simulink library "HDL_ieee_8021513"  (R2024a)
settings: Solver=FixedStepDiscrete  StartTime=0.0  StopTime=10.0  RelTol=1e-3
undefined symbols (not defined in the file): Add, axiWidth, CONST, fs, peakDetectorThreshold, peakDetectorWindow, QAM, Shift
libraries: hdlsllib x199, $bdroot x91, whdlutilities x34, whdledac x9, simulink x8, whdlmod x6, dspsigops x5, dsphdlfiltering2 x4, embreciprocals x3, dsphdlsigops2 x2, commhdlcrc x2, dspstat3 x2
(part 5 of 6)

== system HDL_ieee_8021513/full_tx/new_frame_rate_conversion ==
  note: Description:
      | This block "extends" the "end" signal 4 clock cycles, to ensure that the "end" signal can be sampled by the rate transition block.
      | (Otherwise, the "end" signal would be "on" only 1/4th of a cycle, and it can't be ensured that it will be read).
  ctrl_in : Inport
  Delay2 : Delay  DelayLength=1  InitialCondition=0  UseCircularBuffer=on
  Delay3 : Delay  DelayLength=1  InitialCondition=0  UseCircularBuffer=on
  Delay4 : Delay  DelayLength=1  InitialCondition=0  UseCircularBuffer=on
  Logical Operator : Logic  Operator=OR  Inputs=4  IconShape=distinctive  AllPortsSameDT=off  OutDataTypeStr=boolean
  Rate Transition2 : RateTransition  OutPortSampleTime=4/CONST.fPHY
  Sample Control Bus Selector1 : whdlutilities/Sample Control Bus Selector  OutputSignals=start,end,valid
  State Control : StateControl  StateControl=Synchronous
  Terminator2 : Terminator
  Terminator3 : Terminator
  new_frame : Outport  VectorParamsAs1DForOutWhenUnconnected=off
  wires:
  Logical Operator/1 -> Rate Transition2/1
  Sample Control Bus Selector1/3 -> Terminator2/1  "<valid>"
  Delay2/1 -> Logical Operator/2, Delay3/1
  Delay3/1 -> Logical Operator/3, Delay4/1
  Sample Control Bus Selector1/2 -> Logical Operator/1, Delay2/1  "<end>"
  Delay4/1 -> Logical Operator/4
  Sample Control Bus Selector1/1 -> Terminator3/1  "<start>"
  ctrl_in/1 -> Sample Control Bus Selector1/1
  Rate Transition2/1 -> new_frame/1

== system HDL_ieee_8021513/full_tx/new_frame_rate_conversion1 ==
  note: Description:
      | This block "extends" the "end" signal 8 clock cycles, to ensure that the "end" signal can be sampled by the rate transition block.
      | (Otherwise, the "end" signal would be "on" only 1/4th of a cycle, and it can't be ensured that it will be read).
  ctrl_in : Inport
  Delay{1..7} (7 alike) : Delay  DelayLength=1  InitialCondition=0  UseCircularBuffer=on
  Logical Operator : Logic  Operator=OR  Inputs=8  IconShape=distinctive  AllPortsSameDT=off  OutDataTypeStr=boolean
  Rate Transition2 : RateTransition  OutPortSampleTime=4/CONST.fPHY
  Sample Control Bus Selector1 : whdlutilities/Sample Control Bus Selector  OutputSignals=start,end,valid
  State Control : StateControl  StateControl=Synchronous
  Terminator2 : Terminator
  Terminator3 : Terminator
  new_frame : Outport  VectorParamsAs1DForOutWhenUnconnected=off
  wires:
  Logical Operator/1 -> Rate Transition2/1
  Sample Control Bus Selector1/3 -> Terminator2/1  "<valid>"
  Delay2/1 -> Logical Operator/2, Delay3/1
  Delay3/1 -> Logical Operator/3, Delay4/1
  Sample Control Bus Selector1/2 -> Logical Operator/1, Delay2/1  "<end>"
  Delay4/1 -> Logical Operator/8, Delay1/1
  Sample Control Bus Selector1/1 -> Terminator3/1  "<start>"
  ctrl_in/1 -> Sample Control Bus Selector1/1
  Rate Transition2/1 -> new_frame/1
  Delay1/1 -> Logical Operator/7, Delay5/1
  Delay5/1 -> Logical Operator/6, Delay6/1
  Delay6/1 -> Logical Operator/5, Delay7/1
  Delay7/1 -> Logical Operator/4

== system HDL_ieee_8021513/full_tx/store_frame_in_ram ==
  preamble : Inport
  preamble_valid : Inport  Port=2
  channel : Inport  Port=3
  channel_valid : Inport  Port=4
  header : Inport  Port=5
  header_valid : Inport  Port=6
  payload : Inport  Port=7
  payload_valid : Inport  Port=8
  payload_len : Inport  Port=9
  bits_per_subcarrier : Inport  Port=10
  cp_len_in : Inport  Port=11
  ready : Inport  Port=12
  Delay{,1..5} (6 alike) : Delay  DelayLength=1  InitialCondition=0  UseCircularBuffer=on
  Delay6 : Delay  DelayLength=4  InitialCondition=0  UseCircularBuffer=on
  Simple Dual Port RAM : hdlsllib/HDL RAMs/Simple Dual Port RAM  ram_size=CONST.txRAMAddressBitWidth
  State Control : StateControl  StateControl=Synchronous
  read_frame_from_ram : Subsystem
  write_frame_to_ram : Subsystem
  data_out : Outport
  valid_out : Outport  Port=2
  bits_per_subcarrier_out : Outport  Port=3
  init : Outport  Port=4
  new : Outport  Port=5
  cp_len : Outport  Port=6
  new_psdu : Outport  Port=7  VectorParamsAs1DForOutWhenUnconnected=off
  wires:
  Delay6/1 -> Delay5/1
  Delay5/1 -> new_psdu/1
  ready/1 -> read_frame_from_ram/5(ready)
  Delay4/1 -> cp_len/1
  Delay3/1 -> new/1
  Delay2/1 -> init/1
  Delay1/1 -> bits_per_subcarrier_out/1
  Delay/1 -> valid_out/1
  read_frame_from_ram/3(bits_per_subcarrier_out) -> Delay1/1
  read_frame_from_ram/4(init) -> Delay2/1
  read_frame_from_ram/6(cp_len) -> Delay4/1
  read_frame_from_ram/1(rd_addr) -> Simple Dual Port RAM/4  "new_rd_addr"
  bits_per_subcarrier/1 -> read_frame_from_ram/3(bits_per_subcarrier)
  header/1 -> write_frame_to_ram/5(header)
  write_frame_to_ram/1(write_data) -> Simple Dual Port RAM/1  "new_din"
  write_frame_to_ram/4(end) -> read_frame_from_ram/1(start_reading), Delay6/1
  cp_len_in/1 -> read_frame_from_ram/4(cp_len_in)
  write_frame_to_ram/3(we) -> Simple Dual Port RAM/3  "new_we"
  preamble/1 -> write_frame_to_ram/1(preamble)
  channel_valid/1 -> write_frame_to_ram/4(channel_valid)
  payload/1 -> write_frame_to_ram/7(payload)
  Simple Dual Port RAM/1 -> data_out/1
  read_frame_from_ram/5(new) -> Delay3/1  "new_new"
  write_frame_to_ram/5(ram_size) -> read_frame_from_ram/2(ram_size)
  preamble_valid/1 -> write_frame_to_ram/2(preamble_valid)
  payload_len/1 -> write_frame_to_ram/9(payload_len)
  channel/1 -> write_frame_to_ram/3(channel)
  write_frame_to_ram/2(wr_addr) -> Simple Dual Port RAM/2  "new_wr_addr"
  read_frame_from_ram/2(valid_out) -> Delay/1  "valid_new"
  payload_valid/1 -> write_frame_to_ram/8(payload_valid)
  header_valid/1 -> write_frame_to_ram/6(header_valid)

== system HDL_ieee_8021513/ldpc_encoder/output_selector ==
  codeRate : Inport
  blockSize : Inport  Port=2
  Buffer1 : $bdroot/Buffer  SystemSampleTime=-1  VariantActivationTime=update diagram  AllowFlexibleInterface=on  Latency=0  AutoFrameSizeCalculation=off
  Demux2 : Demux  Outputs=2
  Demux3 : Demux  Outputs=3
  Logical Operator3 : Logic  IconShape=distinctive  AllPortsSameDT=off  OutDataTypeStr=boolean
  Logical Operator5 : Logic  Operator=OR  IconShape=distinctive  AllPortsSameDT=off  OutDataTypeStr=boolean
  Logical Operator6 : Logic  IconShape=distinctive  AllPortsSameDT=off  OutDataTypeStr=boolean
  Logical Operator7 : Logic  Operator=NOT  IconShape=distinctive  AllPortsSameDT=off  OutDataTypeStr=boolean
  Terminator1 : Terminator
  m2 : Outport  VectorParamsAs1DForOutWhenUnconnected=off
  m1 : Outport  Port=2  VectorParamsAs1DForOutWhenUnconnected=off
  m0 : Outport  Port=3  VectorParamsAs1DForOutWhenUnconnected=off
  wires:
  Buffer1/1 -> m0/1  "Out0"
  Logical Operator6/1 -> m1/1  "Out1"
  codeRate/1 -> Demux3/1
  blockSize/1 -> Demux2/1
  Demux2/1 -> Buffer1/1  "K0"
  Demux3/1 -> Logical Operator3/2, Logical Operator7/1  "R0"
  Logical Operator5/1 -> m2/1  "Out2"
  Logical Operator7/1 -> Logical Operator6/1
  Demux3/2 -> Logical Operator6/2, Logical Operator3/1  "R1"
  Demux2/2 -> Terminator1/1  "K1"
  Logical Operator3/1 -> Logical Operator5/1
  Demux3/3 -> Logical Operator5/2  "R2"

== system HDL_ieee_8021513/ofdm_separator/wait_for_header ==
  note: Store payload OFDM symbols until header parameters are known (cyclic prefix has to be known before demodulating the OFDM symbol)
  note: The RAM value should be large enough to wait for the header to be processed.
      | Th e LDPC decoder of the header has a delay > 2500, so a value of 3000 is chosen for an extra margin.
  data_in : Inport
  header_ready : Inport  Port=2
  valid_payload : Inport  Port=3
  zero_payload : Inport  Port=4
  one_payload : Inport  Port=5
  ofdm_samples : Inport  Port=6
  AND : Logic  IconShape=distinctive  AllPortsSameDT=off  OutDataTypeStr=boolean
  Delay12 : Delay  DelayLength=1  InitialCondition=0  UseCircularBuffer=on
  Delay13 : Delay  DelayLength=1  InitialCondition=0  UseCircularBuffer=on
  Delay14 : Delay  DelayLength=1  InitialCondition=0  UseCircularBuffer=on
  HDL Counter : hdlsllib/Sources/HDL Counter  CountType=Free running  CountInit=0  CountStep=1  CountMax=25  CountFromType=Initial value  CountFrom=0  CountResetPort=on  CountLoadPort=off  CountEnbPort=on  CountDirPort=off  CountHitOutputPort=off  CountDataType=Unsigned  CountWordLen=16  CountFracLen=0  CountSampTime=1
  HDL FIFO : hdlsllib/HDL RAMs/HDL FIFO  fifo_size=CONST.FIFOOFDMSize  mode=Classic  ratio=1  push_msg=Error  pop_msg=Error  show_empty=on  show_full=off  show_num=on  LabelModeActiveChoice_Mode=Classic  rst_port=on
  Logical Operator1 : Logic  Operator=OR  Inputs=3  IconShape=distinctive  AllPortsSameDT=off  OutDataTypeStr=boolean
  NOT : Logic  Operator=NOT  IconShape=distinctive  AllPortsSameDT=off  OutDataTypeStr=boolean
  OR : Logic  Operator=OR  IconShape=distinctive  AllPortsSameDT=off  OutDataTypeStr=boolean
  OR2 : Logic  Operator=OR  IconShape=distinctive  AllPortsSameDT=off  OutDataTypeStr=boolean
  Relational Operator : RelationalOperator  Operator===  OutDataTypeStr=boolean  RndMeth=Simplest  InputSameDT=off
  Switch : Switch  Criteria=u2 ~= 0  SaturateOnIntegerOverflow=off  InputSameDT=off
  Switch3 : Switch  Criteria=u2 ~= 0  SaturateOnIntegerOverflow=off  InputSameDT=off
  Terminator : Terminator
  Unit Delay : UnitDelay  SampleTime=-1  HasFrameUpgradeWarning=on
  rising_edge_detector : $bdroot/rising_edge_detector  SystemSampleTime=-1  VariantActivationTime=update diagram  AllowFlexibleInterface=on  Latency=0  AutoFrameSizeCalculation=off
  rising_edge_detector1 : $bdroot/rising_edge_detector  SystemSampleTime=-1  VariantActivationTime=update diagram  AllowFlexibleInterface=on  Latency=0  AutoFrameSizeCalculation=off
  data_out : Outport
  valid_payload_out : Outport  Port=2
  wires:
  Delay13/1 -> HDL FIFO/2
  data_in/1 -> Switch3/3, Delay12/1
  Delay12/1 -> HDL FIFO/1
  valid_payload/1 -> Delay13/1, rising_edge_detector1/1
  Switch3/1 -> data_out/1
  HDL FIFO/2 -> [empty]
  HDL FIFO/1 -> Switch3/1
  rising_edge_detector1/1 -> OR/1
  zero_payload/1 -> OR/2
  HDL FIFO/3 -> Terminator/1  "fifo_ofdm"
  [empty] -> rising_edge_detector/1
  rising_edge_detector/1 -> Logical Operator1/1
  Unit Delay/1 -> Switch/3
  Switch/1 -> Delay14/1, HDL FIFO/3, Unit Delay/1  "pop"
  Logical Operator1/1 -> Switch/2
  header_ready/1 -> HDL Counter/1, Switch/1, Logical Operator1/2
  HDL Counter/1 -> Relational Operator/1  "count"
  ofdm_samples/1 -> Relational Operator/2
  OR/1 -> OR2/1
  Relational Operator/1 -> OR2/2, NOT/1, Logical Operator1/3  "hit_zero"
  OR2/1 -> HDL FIFO/4
  one_payload/1 -> HDL Counter/2
  AND/1 -> Switch3/2, valid_payload_out/1
  Delay14/1 -> AND/1
  NOT/1 -> AND/2

== system HDL_ieee_8021513/ofdm_symbol_sync/find_peak ==
  data_in : Inport
  M_in : Inport  Port=2
  Compare To Constant : hdlsllib/Logic and Bit Operations/Compare To Constant  relop=>  const=CONST.peakDetectorThreshold  OutDataTypeStr=boolean
  Constant : Constant  Value=0  OutDataTypeStr=Inherit: Inherit via back propagation  SampleTime=-1
  Delay{,1..4} (5 alike) : Delay  DelayLength=1  InitialCondition=0  UseCircularBuffer=on
  Delay5 : Delay  DelayLength=CONST.peakDetectorWindow-1  InitialCondition=0  UseCircularBuffer=on
  HDL Counter : hdlsllib/Sources/HDL Counter  CountType=Count limited  CountInit=0  CountStep=1  CountMax=CONST.peakDetectorWindow-1  CountFromType=Initial value  CountFrom=0  CountResetPort=on  CountLoadPort=off  CountEnbPort=on  CountDirPort=off  CountHitOutputPort=on  CountDataType=Unsigned  CountWordLen=nextpow2(CONST.peakDetectorWindow)  CountFracLen=0  CountSampTime=1
  OR : Logic  Operator=OR  IconShape=distinctive  AllPortsSameDT=off  OutDataTypeStr=boolean
  OR1 : Logic  Operator=OR  IconShape=distinctive  AllPortsSameDT=off  OutDataTypeStr=boolean
  Relational Operator : RelationalOperator  Operator=>  OutDataTypeStr=boolean  InputSameDT=off
  Switch : Switch  Criteria=u2 ~= 0  SaturateOnIntegerOverflow=off
  Switch1 : Switch  Criteria=u2 ~= 0  SaturateOnIntegerOverflow=off
  Switch2 : Switch  Criteria=u2 ~= 0  SaturateOnIntegerOverflow=off  InputSameDT=off
  Terminator : Terminator
  Unit Delay : UnitDelay  SampleTime=-1  HasFrameUpgradeWarning=on
  Unit Delay1 : UnitDelay  SampleTime=-1  HasFrameUpgradeWarning=on
  data_out : Outport  VectorParamsAs1DForOutWhenUnconnected=off
  peak_sync : Outport  Port=2  VectorParamsAs1DForOutWhenUnconnected=off
  wires:
  M_in/1 -> Switch1/1, Compare To Constant/1  "data_in"
  Unit Delay/1 -> Switch/3
  Switch/1 -> Unit Delay/1, Relational Operator/2  "peak(i)"
  Relational Operator/1 -> HDL Counter/1, Delay3/1  "new_peak"
  Switch1/1 -> Delay2/1  "peak(i+1)"
  Constant/1 -> Switch1/3
  Unit Delay1/1 -> Switch2/3
  Switch2/1 -> Unit Delay1/1, HDL Counter/2  "en"
  HDL Counter/2 -> Delay1/1, peak_sync/1
  OR/1 -> Switch2/2
  [new_peak] -> OR/2
  [peak_found] -> OR/1
  HDL Counter/1 -> Terminator/1
  Delay/1 -> Switch/1
  Delay1/1 -> [peak_found]  "peak_found"
  OR1/1 -> Switch/2
  [new_peak] -> OR1/1
  [peak_found] -> OR1/2
  Delay3/1 -> [new_peak], Switch2/1
  Compare To Constant/1 -> Switch1/2
  Delay2/1 -> Delay/1, Relational Operator/1
  data_in/1 -> Delay4/1
  Delay4/1 -> Delay5/1
  Delay5/1 -> data_out/1

== system HDL_ieee_8021513/ofdm_symbol_sync/m_cox ==
  note: Delay of m_cox = delay blocks + delay divider + delay_10_preambles_symbols
      | Delay of m_cox = 12 + 47 + 2580
  data_in : Inport
  Compare To Constant : hdlsllib/Logic and Bit Operations/Compare To Constant  relop=>=  const=1  OutDataTypeStr=boolean
  Constant : Constant  OutDataTypeStr=boolean  SampleTime=-1
  Constant1 : Constant  OutDataTypeStr=Inherit: Inherit via back propagation  SampleTime=-1
  Data Type Conversion : DataTypeConversion  OutDataTypeStr=CONST.rxPDataType  SaturateOnIntegerOverflow=off  RndMeth=Floor
  Data Type Conversion1 : DataTypeConversion  OutDataTypeStr=CONST.rxOFDMSSInputDataType  SaturateOnIntegerOverflow=off  RndMeth=Floor
  Data Type Conversion2 : DataTypeConversion  OutDataTypeStr=fixdt(0, CONST.rxRWordLength, CONST.rxRFractionLength)  SaturateOnIntegerOverflow=off  RndMeth=Floor
  Data Type Conversion3 : DataTypeConversion  OutDataTypeStr=fixdt(0, CONST.rxRWordLength, CONST.rxRFractionLength)  SaturateOnIntegerOverflow=off  RndMeth=Floor
  Delay1 : Delay  DelayLength=CONST.rxRDividerDelay  InitialCondition=0  UseCircularBuffer=on
  Delay4 : Delay  DelayLength=(CONST.N+CONST.preambleCyclicPrefixLen)*10+12+CONST.rxRDividerDelay  InitialCondition=0  UseCircularBuffer=on
  Real Divide HDL Optimized : embreciprocals/Real Divide HDL Optimized  OutputType=CONST.rxMDataType
      settings: LibrarySourceBlock=embeddedMatrixLib/Math Operations/Real Divide HDL Optimized
  Switch : Switch  Criteria=u2 ~= 0  SaturateOnIntegerOverflow=off  InputSameDT=off
  Terminator : Terminator
  calculate_P : Subsystem
  calculate_R : Subsystem
  data_out : Outport  VectorParamsAs1DForOutWhenUnconnected=off
  M(d) : Outport  Port=2  VectorParamsAs1DForOutWhenUnconnected=off
  P(d) : Outport  Port=3  VectorParamsAs1DForOutWhenUnconnected=off
  wires:
  Data Type Conversion1/1 -> calculate_P/1(r(d)), calculate_R/1(r(d))
  Data Type Conversion3/1 -> Real Divide HDL Optimized/2
  Data Type Conversion2/1 -> Real Divide HDL Optimized/1
  data_in/1 -> Delay4/1, Data Type Conversion1/1
  Data Type Conversion/1 -> Delay1/1
  Constant/1 -> Real Divide HDL Optimized/3
  calculate_P/1(|P(d)|2) -> Data Type Conversion2/1  "p_sig"
  Real Divide HDL Optimized/1 -> M(d)/1  "M"
  Delay1/1 -> P(d)/1
  Delay4/1 -> data_out/1
  calculate_P/2(P(d)) -> Data Type Conversion/1  "p_pelado"
  Real Divide HDL Optimized/2 -> Terminator/1
  Constant1/1 -> Switch/3
  Compare To Constant/1 -> Switch/2
  Switch/1 -> Data Type Conversion3/1
  calculate_R/1(Rf2) -> Switch/1, Compare To Constant/1  "r_sig"

== system HDL_ieee_8021513/ofdm_symbol_sync/phase_offset_calculator ==
  peak_sync : Inport
  P(d) : Inport  Port=2
  Complex to Magnitude-Angle : dsphdlmathfun2/Complex to Magnitude-Angle  NumIterationsSource=Auto  NumIterations=10  OutputFormat=Angle  AngleFormat=Normalized  ScaleOutput=off  ScalingMethod=Shift-Add  SimulateUsing=Code generation
  Data Type Conversion : DataTypeConversion  OutDataTypeStr=CONST.rxPhaseDataType  SaturateOnIntegerOverflow=off  RndMeth=Floor
  Delay2 : Delay  InitialCondition=0  UseCircularBuffer=on
  Delay3 : Delay  InitialCondition=0  UseCircularBuffer=on
  Switch : Switch  Criteria=u2 ~= 0  SaturateOnIntegerOverflow=off  InputSameDT=off
  Unit Delay : UnitDelay  SampleTime=-1  HasFrameUpgradeWarning=on
  frequency_offset : Outport
  wires:
  Data Type Conversion/1 -> Delay2/1
  Switch/1 -> Unit Delay/1, frequency_offset/1
  Unit Delay/1 -> Switch/3
  Delay2/1 -> Switch/1
  Delay3/1 -> Switch/2
  Complex to Magnitude-Angle/1 -> Data Type Conversion/1
  P(d)/1 -> Complex to Magnitude-Angle/1
  peak_sync/1 -> Complex to Magnitude-Angle/2
  Complex to Magnitude-Angle/2 -> Delay3/1

== system HDL_ieee_8021513/peak_detector/local_peak ==
  index : Inport
  dataIn : Inport  Port=2
  AND : Logic  IconShape=distinctive  AllPortsSameDT=off  OutDataTypeStr=boolean
  AND1 : Logic  IconShape=distinctive  AllPortsSameDT=off  OutDataTypeStr=boolean
  AND2 : Logic  IconShape=distinctive  AllPortsSameDT=off  OutDataTypeStr=boolean
  Delay{,1..5} (6 alike) : Delay  DelayLength=1  InitialCondition=0  UseCircularBuffer=on
  HDL Counter : hdlsllib/Sources/HDL Counter  CountType=Count limited  CountInit=0  CountStep=1  CountMax=peakDetectorWindow-1  CountFromType=Initial value  CountFrom=0  CountResetPort=on  CountLoadPort=off  CountEnbPort=on  CountDirPort=off  CountHitOutputPort=on  CountDataType=Unsigned  CountWordLen=nextpow2(peakDetectorWindow+1)  CountFracLen=0  CountSampTime=-1
  NOT : Logic  Operator=NOT  IconShape=distinctive  AllPortsSameDT=off  OutDataTypeStr=boolean
  OR : Logic  Operator=OR  IconShape=distinctive  AllPortsSameDT=off  OutDataTypeStr=boolean
  OR1 : Logic  Operator=OR  IconShape=distinctive  AllPortsSameDT=off  OutDataTypeStr=boolean
  OR2 : Logic  Operator=OR  IconShape=distinctive  AllPortsSameDT=off  OutDataTypeStr=boolean
  Relational Operator : RelationalOperator  OutDataTypeStr=boolean  RndMeth=Simplest  InputSameDT=off
  Switch : Switch  Criteria=u2 ~= 0  SaturateOnIntegerOverflow=off  InputSameDT=off
  Switch1 : Switch  Criteria=u2 ~= 0  SaturateOnIntegerOverflow=off  InputSameDT=off
  Terminator : Terminator
  Unit Delay : UnitDelay  SampleTime=-1  HasFrameUpgradeWarning=on
  Unit Delay1 : UnitDelay  SampleTime=-1  HasFrameUpgradeWarning=on
  peak_sync : Outport
  wires:
  HDL Counter/1 -> Terminator/1  "count"
  Unit Delay/1 -> Switch/3
  Switch/1 -> Relational Operator/2, Unit Delay/1  "dataIn(indexes(i)"
  Unit Delay1/1 -> Switch1/3
  Switch1/1 -> HDL Counter/2, Delay3/1, Unit Delay1/1  "count_enable"
  OR/1 -> Delay4/1
  dataIn/1 -> Relational Operator/1, Delay1/1
  index/1 -> AND1/1  "input"
  Delay4/1 -> Switch1/2  "open"
  Delay5/1 -> Switch1/1  "new_index"
  Delay/1 -> Switch/2
  Delay1/1 -> Switch/1
  Relational Operator/1 -> [higher]
  NOT/1 -> AND1/2
  AND1/1 -> [new_peak], OR1/1
  OR1/1 -> Delay2/1  "rst"
  AND2/1 -> OR1/2
  AND/1 -> OR2/1
  OR2/1 -> Delay/1
  [en] -> NOT/1
  [en] -> AND2/1
  [en] -> AND/1
  Delay3/1 -> [en]
  [higher] -> AND/2
  [higher] -> AND2/2
  [peak_found] -> OR/2
  HDL Counter/2 -> peak_sync/1, [peak_found]  "counter_hit"
  [new_peak] -> Delay5/1
  [new_peak] -> OR/1
  [new_peak] -> OR2/2
  Delay2/1 -> HDL Counter/1  "new_index"

== system HDL_ieee_8021513/peak_detector/s1_index ==
  dataIn : Inport
  Add : Sum
  Bit Shift : hdlsllib/Logic and Bit Operations/Bit Shift  mode=Shift Right Arithmetic  N=1
  Compare To Constant : hdlsllib/Logic and Bit Operations/Compare To Constant  relop=>  const=peakDetectorThreshold  OutDataTypeStr=boolean
  Delay : Delay  DelayLength=peakDetectorWindow  InitialCondition=0  UseCircularBuffer=on
  Delay{1..5} (5 alike) : Delay  DelayLength=1  InitialCondition=0  UseCircularBuffer=on
  Minimum : dspstat3/Minimum  operation=minimum  fcn=Value  indexBase=Zero  operateOver=Each column  Dimension=1  InputProcessing=Columns as channels (frame based)  reset=None  roiEnable=off  roiType=Rectangles  roiPortion=Entire ROI  roiOutput=Individual statistics for each ROI  roiFlag=off  roundingMode=Floor  overflowMode=off
      settings: LibrarySourceBlock=dsphdlsupportstat/Minimum
  Minimum1 : dspstat3/Minimum  operation=minimum  fcn=Value  indexBase=Zero  operateOver=Each column  Dimension=1  InputProcessing=Columns as channels (frame based)  reset=None  roiEnable=off  roiType=Rectangles  roiPortion=Entire ROI  roiOutput=Individual statistics for each ROI  roiFlag=off  roundingMode=Floor  overflowMode=off
      settings: LibrarySourceBlock=dsphdlsupportstat/Minimum
  Tapped Delay : simulink/Discrete/Tapped Delay  vinit=0.0  samptime=-1  NumDelays=peakDetectorWindow  DelayOrder=Oldest  includeCurrent=off
  Tapped Delay1 : simulink/Discrete/Tapped Delay  vinit=0.0  samptime=-1  NumDelays=peakDetectorWindow  DelayOrder=Oldest  includeCurrent=off
  indexes : Outport
  Output : Outport  Port=2
  wires:
  dataIn/1 -> Tapped Delay/1, Delay/1  "x(i+peakDetectorWindow+1)"
  Delay/1 -> Delay2/1  "x(i+1)"
  Tapped Delay/1 -> Minimum/1  "x(i+1:i+peakDetectorWindow)"
  Tapped Delay1/1 -> Minimum1/1  "x(i-peakDetectorWindow:i-1)"
  Minimum/1 -> Add/1  "xmin_new"
  Minimum1/1 -> Add/2  "xmin_bot"
  Bit Shift/1 -> Delay3/1  "s1"
  Delay2/1 -> Delay4/1, Tapped Delay1/1  "x(i)"
  Compare To Constant/1 -> indexes/1
  Add/1 -> Delay1/1
  Delay1/1 -> Bit Shift/1
  Delay3/1 -> Compare To Constant/1
  Delay4/1 -> Delay5/1
  Delay5/1 -> Output/1

== system HDL_ieee_8021513/qam_demod/to_12bit_integer ==
  1bit : Inport
  2bit : Inport  Port=2
  4bit : Inport  Port=3
  Constant{,1..2,12,14} (5 alike) : Constant  Value=0  OutDataTypeStr=Inherit: Inherit via back propagation  SampleTime=-1
  Demux : Demux  Outputs=2
  Demux1 : Demux
  Vector Concatenate : Concatenate  NumInputs=4  Mode=Multidimensional array
  Vector Concatenate1 : Concatenate  NumInputs=4  Mode=Multidimensional array
  Vector Concatenate2 : Concatenate  NumInputs=4  Mode=Multidimensional array
  1bit_out : Outport
  2bit_out : Outport  Port=2
  4bit_out : Outport  Port=3
  wires:
  2bit/1 -> Demux/1
  4bit/1 -> Demux1/1
  Vector Concatenate/1 -> 4bit_out/1
  Vector Concatenate1/1 -> 2bit_out/1
  Vector Concatenate2/1 -> 1bit_out/1
  Constant2/1 -> Vector Concatenate2/1
  Constant1/1 -> Vector Concatenate2/2
  Constant/1 -> Vector Concatenate2/3
  1bit/1 -> Vector Concatenate2/4
  Constant14/1 -> Vector Concatenate1/1
  Constant12/1 -> Vector Concatenate1/2
  Demux/1 -> Vector Concatenate1/3
  Demux/2 -> Vector Concatenate1/4
  Demux1/1 -> Vector Concatenate/1
  Demux1/2 -> Vector Concatenate/2
  Demux1/3 -> Vector Concatenate/3
  Demux1/4 -> Vector Concatenate/4

== system HDL_ieee_8021513/rx_demodulator_full/get_bits_per_subcarrier ==
  payload_bits_per_sub : Inport
  valid_header : Inport  Port=2
  Constant3 : Constant  Value=CONST.headerBitsPerSubcarrier  OutDataTypeStr=uint8  SampleTime=-1
  Data Type Conversion2 : DataTypeConversion  OutDataTypeStr=fixdt(0,4,0)  SaturateOnIntegerOverflow=off  RndMeth=Floor
  Data Type Conversion7 : DataTypeConversion  OutDataTypeStr=fixdt(0,4,0)  SaturateOnIntegerOverflow=off  RndMeth=Floor
  Switch1 : Switch  Criteria=u2 ~= 0  SaturateOnIntegerOverflow=off  InputSameDT=off
  qam_demod_bits : Outport
  wires:
  Data Type Conversion7/1 -> Switch1/1
  Constant3/1 -> Data Type Conversion7/1
  Data Type Conversion2/1 -> Switch1/3
  valid_header/1 -> Switch1/2
  payload_bits_per_sub/1 -> Data Type Conversion2/1
  Switch1/1 -> qam_demod_bits/1

== system HDL_ieee_8021513/rx_demodulator_full/get_cp ==
  valid_header : Inport
  valid_payload : Inport  Port=2
  cp_payload : Inport  Port=3
  Bit Concat : hdlsllib/Logic and Bit Operations/Bit Concat  numInputs=2
  Constant : Constant  Value=CONST.channelCyclicPrefixLen  OutDataTypeStr=uint8  SampleTime=-1
  Constant1 : Constant  Value=CONST.headerCyclicPrefixLen  OutDataTypeStr=uint8  SampleTime=-1
  Data Type Conversion : DataTypeConversion  OutDataTypeStr=uint8  SaturateOnIntegerOverflow=off  RndMeth=Floor
  Data Type Conversion1 : DataTypeConversion  OutDataTypeStr=fixdt(0,2,0)  SaturateOnIntegerOverflow=off  RndMeth=Floor
  Data Type Conversion5 : DataTypeConversion  OutDataTypeStr=uint8  SaturateOnIntegerOverflow=off  RndMeth=Floor
  Data Type Conversion6 : DataTypeConversion  OutDataTypeStr=uint8  SaturateOnIntegerOverflow=off  RndMeth=Floor
  Multiport Switch : MultiPortSwitch  DataPortOrder=Zero-based contiguous  zeroidx=on  SaturateOnIntegerOverflow=off
  ofdm_cp_len : Outport
  wires:
  Bit Concat/1 -> Data Type Conversion1/1  "control"
  Constant1/1 -> Data Type Conversion5/1
  Constant/1 -> Data Type Conversion6/1
  cp_payload/1 -> Data Type Conversion/1
  Multiport Switch/1 -> ofdm_cp_len/1
  Data Type Conversion6/1 -> Multiport Switch/2
  Data Type Conversion5/1 -> Multiport Switch/3
  Data Type Conversion/1 -> Multiport Switch/4
  valid_payload/1 -> Bit Concat/1
  valid_header/1 -> Bit Concat/2
  Data Type Conversion1/1 -> Multiport Switch/1

== system HDL_ieee_8021513/rx_demodulator_full/get_init ==
  valid_header : Inport
  valid_payload : Inport  Port=2
  Bit Concat : hdlsllib/Logic and Bit Operations/Bit Concat  numInputs=2
  Constant4 : Constant  Value=CONST.channelScramblerInit  OutDataTypeStr=uint8  SampleTime=-1
  Constant5 : Constant  Value=CONST.headerScramblerInit  OutDataTypeStr=uint8  SampleTime=-1
  Constant6 : Constant  Value=CONST.payloadScramblerInit  OutDataTypeStr=uint8  SampleTime=-1
  Data Type Conversion10 : DataTypeConversion  OutDataTypeStr=boolean  SaturateOnIntegerOverflow=off  RndMeth=Floor
  Data Type Conversion4 : DataTypeConversion  OutDataTypeStr=boolean  SaturateOnIntegerOverflow=off  RndMeth=Floor
  Data Type Conversion9 : DataTypeConversion  OutDataTypeStr=boolean  SaturateOnIntegerOverflow=off  RndMeth=Floor
  Multiport Switch2 : MultiPortSwitch  DataPortOrder=Zero-based contiguous  zeroidx=on  SaturateOnIntegerOverflow=off  InputSameDT=off
  descrambler_init : Outport
  wires:
  Data Type Conversion9/1 -> Multiport Switch2/3
  Constant6/1 -> Data Type Conversion4/1
  Data Type Conversion4/1 -> Multiport Switch2/4
  Constant5/1 -> Data Type Conversion9/1
  Constant4/1 -> Data Type Conversion10/1
  Multiport Switch2/1 -> descrambler_init/1
  Data Type Conversion10/1 -> Multiport Switch2/2
  valid_payload/1 -> Bit Concat/1
  valid_header/1 -> Bit Concat/2
  Bit Concat/1 -> Multiport Switch2/1  "control"

== system HDL_ieee_8021513/rx_demodulator_full/ofdm_rx_counter ==
  note: Counts the amount of OFDM symbols for every "end" signal, and assigns them a position (preamble, channel, header, payload)
  valid : Inport
  rst : Inport  Port=2
  payload_num_ofdm_symbols : Inport  Port=3
  Add : Sum
  Constant1 : Constant  Value=2  OutDataTypeStr=uint16  SampleTime=-1
  Constant2 : Constant  Value=3  OutDataTypeStr=uint16  SampleTime=-1
  Constant3 : Constant  Value=3  OutDataTypeStr=uint16  SampleTime=-1
  HDL Counter : hdlsllib/Sources/HDL Counter  CountType=Free running  CountInit=0  CountStep=1  CountMax=25  CountFromType=Initial value  CountFrom=0  CountResetPort=on  CountLoadPort=off  CountEnbPort=on  CountDirPort=off  CountHitOutputPort=off  CountDataType=Unsigned  CountWordLen=16  CountFracLen=0  CountSampTime=1
  Logical Operator2 : Logic  IconShape=distinctive  AllPortsSameDT=off  OutDataTypeStr=boolean
  Logical Operator3 : Logic  Operator=NOT  IconShape=distinctive  AllPortsSameDT=off  OutDataTypeStr=boolean
  Logical Operator4 : Logic  Operator=NOT  IconShape=distinctive  AllPortsSameDT=off  OutDataTypeStr=boolean
  Logical Operator5 : Logic  IconShape=distinctive  AllPortsSameDT=off  OutDataTypeStr=boolean
  Relational Operator1 : RelationalOperator  Operator=<  OutDataTypeStr=boolean  InputSameDT=off
  Relational Operator2 : RelationalOperator  Operator=<  OutDataTypeStr=boolean  InputSameDT=off
  Relational Operator3 : RelationalOperator  Operator=<  OutDataTypeStr=boolean  InputSameDT=off
  falling_edge_detector : $bdroot/falling_edge_detector  SystemSampleTime=-1  VariantActivationTime=update diagram  AllowFlexibleInterface=on  Latency=0  AutoFrameSizeCalculation=off
  falling_edge_detector1 : $bdroot/falling_edge_detector  SystemSampleTime=-1  VariantActivationTime=update diagram  AllowFlexibleInterface=on  Latency=0  AutoFrameSizeCalculation=off
  rising_edge_detector1 : $bdroot/rising_edge_detector  SystemSampleTime=-1  VariantActivationTime=update diagram  AllowFlexibleInterface=on  Latency=0  AutoFrameSizeCalculation=off
  is_channel : Outport
  is_header : Outport  Port=2
  is_payload : Outport  Port=3
  last_frame : Outport  Port=4  VectorParamsAs1DForOutWhenUnconnected=off
  wires:
  rising_edge_detector1/1 -> HDL Counter/1
  rst/1 -> rising_edge_detector1/1
  Relational Operator1/1 -> is_channel/1, Logical Operator3/1  "channel"
  Logical Operator2/1 -> is_header/1  "header"
  Logical Operator3/1 -> Logical Operator2/1
  Relational Operator2/1 -> Logical Operator2/2, Logical Operator4/1
  HDL Counter/1 -> Relational Operator3/1, Relational Operator2/1, Relational Operator1/1
  Constant2/1 -> Relational Operator2/2
  Constant1/1 -> Relational Operator1/2
  falling_edge_detector1/1 -> HDL Counter/2
  valid/1 -> falling_edge_detector1/1
  Logical Operator4/1 -> Logical Operator5/1  "payload"
  Logical Operator5/1 -> falling_edge_detector/1, is_payload/1  "payload"
  falling_edge_detector/1 -> last_frame/1
  payload_num_ofdm_symbols/1 -> Add/2
  Add/1 -> Relational Operator3/2
  Constant3/1 -> Add/1
  Relational Operator3/1 -> Logical Operator5/2

== system HDL_ieee_8021513/rx_payload_full/data_words_in_payload ==
  note: Remove excess words as indicated in msg_duration
  psdu_size : Inport
  msg_duration : Inport  Port=2
  Bits to Word : hdlsllib/Logic and Bit Operations/Bits to Word
  Bits to Word1 : hdlsllib/Logic and Bit Operations/Bits to Word
  Data Type Conversion : DataTypeConversion  OutDataTypeStr=fixdt(0,1,0)  SaturateOnIntegerOverflow=off  RndMeth=Floor
  Data Type Conversion1 : DataTypeConversion  OutDataTypeStr=fixdt(0,1,0)  SaturateOnIntegerOverflow=off  RndMeth=Floor
  Delay : Delay  DelayLength=1  InitialCondition=0  UseCircularBuffer=on
  Subtract : Sum  Inputs=+-
  payload_words : Outport
  wires:
  Subtract/1 -> Delay/1
  Delay/1 -> payload_words/1
  Bits to Word1/1 -> Subtract/2
  Bits to Word/1 -> Subtract/1
  msg_duration/1 -> Data Type Conversion1/1
  Data Type Conversion1/1 -> Bits to Word1/1
  psdu_size/1 -> Data Type Conversion/1
  Data Type Conversion/1 -> Bits to Word/1

== system HDL_ieee_8021513/rx_payload_full/next_frame_to_ready_rx ==
  note: Given a next frame rising edge, this subsystem will generate a "ready" signal for the duration of "payloadBitsPerFec" clock cycles
  next_frame : Inport
  HDL Counter : hdlsllib/Sources/HDL Counter  CountType=Count limited  CountInit=0  CountStep=1  CountMax=CONST.payloadBitsPerFec-1  CountFromType=Initial value  CountFrom=0  CountResetPort=off  CountLoadPort=off  CountEnbPort=on  CountDirPort=off  CountHitOutputPort=on  CountDataType=Unsigned  CountWordLen=nextpow2(CONST.payloadBitsPerFec)  CountFracLen=0  CountSampTime=1
  Logical Operator2 : Logic  Operator=NOT  IconShape=distinctive  AllPortsSameDT=off  OutDataTypeStr=boolean
  Logical Operator3 : Logic  Operator=OR  IconShape=distinctive  AllPortsSameDT=off  OutDataTypeStr=boolean
  Terminator : Terminator
  Unit Delay Enabled Synchronous : hdlsllib/Discrete/Unit Delay Enabled Synchronous  InitialCondition=0.0  SampleTime=-1
  rising_edge_detector : $bdroot/rising_edge_detector  SystemSampleTime=-1  VariantActivationTime=update diagram  AllowFlexibleInterface=on  Latency=0  AutoFrameSizeCalculation=off
  ready : Outport  VectorParamsAs1DForOutWhenUnconnected=off
  wires:
  rising_edge_detector/1 -> Logical Operator3/1
  Logical Operator2/1 -> Unit Delay Enabled Synchronous/1
  HDL Counter/1 -> Terminator/1
  Unit Delay Enabled Synchronous/1 -> HDL Counter/1, ready/1
  Logical Operator3/1 -> Unit Delay Enabled Synchronous/2
  HDL Counter/2 -> Logical Operator3/2, Logical Operator2/1
  next_frame/1 -> rising_edge_detector/1

== system HDL_ieee_8021513/channel_estimation_and_equalization/Channel Equalization/equalizer ==
  data_in : Inport
  hEst : Inport  Port=2
  Valid : Inport  Port=3
  Add : Sum
  Complex to Real-Imag : ComplexToRealImag
  Complex to Real-Imag1 : ComplexToRealImag
  Conjugate : Math  Operator=conj  SignedPower=on  OutputSignalType=complex  RndMeth=Zero
  Data Type Conversion : DataTypeConversion  OutDataTypeStr=fixdt(1,CONST.rxChannelEstReferenceWordLength, CONST.rxChannelEstReferenceFractionLength)  SaturateOnIntegerOverflow=off  RndMeth=Floor
  Data Type Conversion1 : DataTypeConversion  OutDataTypeStr=fixdt(1,CONST.rxChannelEstReferenceWordLength, CONST.rxChannelEstReferenceFractionLength)  SaturateOnIntegerOverflow=off  RndMeth=Floor
  Delay{7..11} (5 alike) : Delay  InitialCondition=0  UseCircularBuffer=on
  Delay13 : Delay  DelayLength=6  InitialCondition=0  UseCircularBuffer=on
  Product : Product
  Product1 : Product
  Real Divide HDL Optimized : embreciprocals/Real Divide HDL Optimized  OutputType=CONST.rxOFDMDemodDataType
      settings: LibrarySourceBlock=embeddedMatrixLib/Math Operations/Real Divide HDL Optimized
  Real Divide HDL Optimized1 : embreciprocals/Real Divide HDL Optimized  OutputType=CONST.rxOFDMDemodDataType
      settings: LibrarySourceBlock=embeddedMatrixLib/Math Operations/Real Divide HDL Optimized
  Real-Imag to Complex : RealImagToComplex
  Terminator : Terminator
  complex_multiplier : $bdroot/complex_multiplier  SystemSampleTime=-1  VariantActivationTime=update diagram  AllowFlexibleInterface=on  Latency=0  AutoFrameSizeCalculation=off
  data_out : Outport
  valid_out : Outport  Port=2
  wires:
  Complex to Real-Imag1/2 -> Real Divide HDL Optimized1/1
  Complex to Real-Imag/2 -> Delay8/1
  Real Divide HDL Optimized/2 -> Terminator/1
  hEst/1 -> Conjugate/1, Complex to Real-Imag/1
  Conjugate/1 -> complex_multiplier/2
  Delay13/1 -> Real Divide HDL Optimized1/3, Real Divide HDL Optimized/3
  Complex to Real-Imag1/1 -> Real Divide HDL Optimized/1
  Delay11/1 -> Data Type Conversion1/1
  Delay7/1 -> Product/2, Product/1
  data_in/1 -> complex_multiplier/1
  Real Divide HDL Optimized1/1 -> Real-Imag to Complex/2
  Complex to Real-Imag/1 -> Delay7/1
  Real-Imag to Complex/1 -> data_out/1
  Product/1 -> Delay10/1
  Add/1 -> Delay11/1
  Real Divide HDL Optimized/1 -> Real-Imag to Complex/1
  Delay8/1 -> Product1/2, Product1/1
  Valid/1 -> Delay13/1
  complex_multiplier/1 -> Data Type Conversion/1
  Data Type Conversion1/1 -> Real Divide HDL Optimized1/2, Real Divide HDL Optimized/2
  Product1/1 -> Delay9/1
  Delay10/1 -> Add/1
  Real Divide HDL Optimized1/2 -> valid_out/1
  Data Type Conversion/1 -> Complex to Real-Imag1/1
  Delay9/1 -> Add/2

== system HDL_ieee_8021513/constellation_descrambler/rotate_-90/rotate_-90 ==
  s2 : Inport
  s1 : Inport  Port=2
  data_in : Inport  Port=3
  Bit Concat : hdlsllib/Logic and Bit Operations/Bit Concat  numInputs=2
  Complex to Real-Imag : ComplexToRealImag
  Complex to Real-Imag1 : ComplexToRealImag
  Complex to Real-Imag2 : ComplexToRealImag
  Multiport Switch : MultiPortSwitch  DataPortOrder=Zero-based contiguous  Inputs=4  zeroidx=on  SaturateOnIntegerOverflow=off  InputSameDT=off
  Real-Imag to Complex : RealImagToComplex
  Real-Imag to Complex1 : RealImagToComplex
  Real-Imag to Complex2 : RealImagToComplex
  Unary Minus{,1..3} (4 alike) : UnaryMinus
  data_out : Outport
  wires:
  Unary Minus3/1 -> Real-Imag to Complex/2
  Multiport Switch/1 -> data_out/1
  Real-Imag to Complex2/1 -> Multiport Switch/5
  Complex to Real-Imag2/1 -> Real-Imag to Complex2/2
  Real-Imag to Complex1/1 -> Multiport Switch/3
  Complex to Real-Imag1/2 -> Real-Imag to Complex1/1
  Real-Imag to Complex/1 -> Multiport Switch/4
  Complex to Real-Imag/2 -> Unary Minus3/1
  Unary Minus/1 -> Real-Imag to Complex/1
  Complex to Real-Imag/1 -> Unary Minus/1
  data_in/1 -> Multiport Switch/2, Complex to Real-Imag/1, Complex to Real-Imag2/1, Complex to Real-Imag1/1
  Bit Concat/1 -> Multiport Switch/1
  s1/1 -> Bit Concat/2
  s2/1 -> Bit Concat/1
  Complex to Real-Imag1/1 -> Unary Minus1/1
  Unary Minus1/1 -> Real-Imag to Complex1/2
  Complex to Real-Imag2/2 -> Unary Minus2/1
  Unary Minus2/1 -> Real-Imag to Complex2/1

== system HDL_ieee_8021513/full_rx/prepare_payload_data/payload_clock_x2 ==
  data_in : Inport
  valid_in : Inport  Port=2
  Serializer1D : hdlsllib/HDL Operations/Serializer1D  Ratio=2  IdleCycles=0  validIn=on  startOut=off  validOut=on  inputDataDimensions=-1  inputSampleTime=-1  inputSignalType=auto
  data_out : Outport
  valid_out : Outport  Port=2
  wires:
  data_in/1 -> Serializer1D/1
  Serializer1D/1 -> data_out/1
  Serializer1D/2 -> valid_out/1
  valid_in/1 -> Serializer1D/2

== system HDL_ieee_8021513/full_tx/store_frame_in_ram/read_frame_from_ram ==
  start_reading : Inport
  ram_size : Inport  Port=2
  bits_per_subcarrier : Inport  Port=3
  cp_len_in : Inport  Port=4
  ready : Inport  Port=5
  AND : Logic  IconShape=distinctive  AllPortsSameDT=off  OutDataTypeStr=boolean
  Compare To Zero1 : hdlsllib/Logic and Bit Operations/Compare To Zero  relop===  OutDataTypeStr=boolean
  Delay{,1..5} (6 alike) : Delay  DelayLength=1  InitialCondition=0  UseCircularBuffer=on
  Delay6 : Delay  InitialCondition=0  UseCircularBuffer=on
  Delay7 : Delay  InitialCondition=0  UseCircularBuffer=on
  HDL Counter1 : hdlsllib/Sources/HDL Counter  CountType=Free running  CountInit=0  CountStep=1  CountMax=1  CountFromType=Initial value  CountFrom=0  CountResetPort=on  CountLoadPort=off  CountEnbPort=on  CountDirPort=off  CountHitOutputPort=off  CountDataType=Unsigned  CountWordLen=CONST.txRAMAddressBitWidth  CountFracLen=0  CountSampTime=1
  HDL Counter2 : hdlsllib/Sources/HDL Counter  CountType=Count limited  CountInit=0  CountStep=1  CountMax=CONST.numDataCarriers-1  CountFromType=Initial value  CountFrom=0  CountResetPort=on  CountLoadPort=off  CountEnbPort=on  CountDirPort=off  CountHitOutputPort=off  CountDataType=Unsigned  CountWordLen=nextpow2(CONST.numDataCarriers)  CountFracLen=0  CountSampTime=1
  Logical Operator4 : Logic  IconShape=distinctive  AllPortsSameDT=off  OutDataTypeStr=boolean
  Logical Operator5 : Logic  Operator=OR  AllPortsSameDT=off  OutDataTypeStr=boolean
  Relational Operator1 : RelationalOperator  Operator===  OutDataTypeStr=boolean  InputSameDT=off
  State Control : StateControl  StateControl=Synchronous
  Switch1 : Switch  Criteria=u2 ~= 0  SaturateOnIntegerOverflow=off  InputSameDT=off
  Unit Delay1 : UnitDelay  SampleTime=-1  HasFrameUpgradeWarning=on
  bits_selector : Subsystem
  cp_len_creator : Subsystem
  init_selector : Subsystem
  rd_addr : Outport  VectorParamsAs1DForOutWhenUnconnected=off
  valid_out : Outport  Port=2  VectorParamsAs1DForOutWhenUnconnected=off
  bits_per_subcarrier_out : Outport  Port=3  VectorParamsAs1DForOutWhenUnconnected=off
  init : Outport  Port=4  VectorParamsAs1DForOutWhenUnconnected=off
  new : Outport  Port=5  VectorParamsAs1DForOutWhenUnconnected=off
  cp_len : Outport  Port=6  VectorParamsAs1DForOutWhenUnconnected=off
  wires:
  ready/1 -> AND/2
  AND/1 -> HDL Counter1/2, Delay7/1
  [rst] -> HDL Counter2/1
  [rst] -> HDL Counter1/1
  Logical Operator4/1 -> Delay1/1
  HDL Counter2/1 -> Compare To Zero1/1
  Compare To Zero1/1 -> Logical Operator4/2
  Delay6/1 -> Delay2/1
  Delay5/1 -> bits_per_subcarrier_out/1
  Delay4/1 -> cp_len/1
  Delay3/1 -> init/1
  Delay2/1 -> rd_addr/1
  Delay1/1 -> new/1
  Delay/1 -> valid_out/1
  Switch1/1 -> Unit Delay1/1, AND/1
  bits_selector/1(bits_per_subcarrier_out) -> Delay5/1
  Unit Delay1/1 -> Switch1/3
  bits_per_subcarrier/1 -> bits_selector/2(bits_per_subcarrier)
  cp_len_creator/1(cp_len) -> Delay4/1
  init_selector/1(init) -> Delay3/1
  Logical Operator5/1 -> Switch1/2
  cp_len_in/1 -> cp_len_creator/2(cp_len_in)
  Relational Operator1/1 -> Logical Operator5/2
  HDL Counter1/1 -> Delay6/1, bits_selector/1(rd_addr), Relational Operator1/2, cp_len_creator/1(rd_addr), init_selector/1(rd_addr)  "rd_addr"
  start_reading/1 -> Logical Operator5/1, Switch1/1, [rst]
  ram_size/1 -> Relational Operator1/1
  Delay7/1 -> HDL Counter2/2, Logical Operator4/1, Delay/1

== system HDL_ieee_8021513/full_tx/store_frame_in_ram/write_frame_to_ram ==
  preamble : Inport
  preamble_valid : Inport  Port=2
  channel : Inport  Port=3
  channel_valid : Inport  Port=4
  header : Inport  Port=5
  header_valid : Inport  Port=6
  payload : Inport  Port=7
  payload_valid : Inport  Port=8
  payload_len : Inport  Port=9
  AND : Logic  IconShape=distinctive  AllPortsSameDT=off  OutDataTypeStr=boolean
  Add1 : Sum
  Compare To Zero : hdlsllib/Logic and Bit Operations/Compare To Zero  relop=~=  OutDataTypeStr=boolean
  Constant43 : Constant  Value=CONST.numDataCarriers  OutDataTypeStr=uint8  SampleTime=-1
  Constant73 : Constant  Value=CONST.preambleDataCarriers + CONST.channelDataCarriers + CONST.headerDataCarriers  OutDataTypeStr=fixdt(0,13,0)  SampleTime=-1
  Delay : Delay  InitialCondition=0  UseCircularBuffer=on
  Delay1 : Delay  InitialCondition=0  UseCircularBuffer=on
  Delay3 : Delay  DelayLength=1  InitialCondition=0  UseCircularBuffer=on
  Delay8 : Delay  InitialCondition=0  UseCircularBuffer=on
  Delay9 : Delay  DelayLength=1  InitialCondition=0  UseCircularBuffer=on
  HDL Counter : hdlsllib/Sources/HDL Counter  CountType=Free running  CountInit=0  CountStep=1  CountMax=1  CountFromType=Initial value  CountFrom=0  CountResetPort=on  CountLoadPort=off  CountEnbPort=on  CountDirPort=off  CountHitOutputPort=off  CountDataType=Unsigned  CountWordLen=CONST.txRAMAddressBitWidth  CountFracLen=0  CountSampTime=1
  Logical Operator : Logic  Operator=OR  Inputs=4  IconShape=distinctive  AllPortsSameDT=off  OutDataTypeStr=boolean
  Product : Product
  Relational Operator : RelationalOperator  Operator===  OutDataTypeStr=boolean  InputSameDT=off
  State Control : StateControl  StateControl=Synchronous
  ram_formatting : Subsystem
  write_data : Outport  VectorParamsAs1DForOutWhenUnconnected=off
  wr_addr : Outport  Port=2  VectorParamsAs1DForOutWhenUnconnected=off
  we : Outport  Port=3  VectorParamsAs1DForOutWhenUnconnected=off
  end : Outport  Port=4  VectorParamsAs1DForOutWhenUnconnected=off
  ram_size : Outport  Port=5  VectorParamsAs1DForOutWhenUnconnected=off
  wires:
  Delay1/1 -> Product/1
  Delay/1 -> Product/2
  AND/1 -> Delay3/1
  Compare To Zero/1 -> AND/2
  Delay3/1 -> end/1, HDL Counter/1  "start_reading"
  channel_valid/1 -> Logical Operator/2, ram_formatting/2(channel_valid)
  header_valid/1 -> Logical Operator/3, ram_formatting/3(header_valid)
  Relational Operator/1 -> AND/1
  Logical Operator/1 -> HDL Counter/2, we/1  "we"
  HDL Counter/1 -> Compare To Zero/1, Relational Operator/2, wr_addr/1  "wr_addr"
  preamble_valid/1 -> ram_formatting/1(preamble_valid), Logical Operator/1
  payload_valid/1 -> Logical Operator/4, ram_formatting/4(payload_valid)
  preamble/1 -> ram_formatting/5(preamble)
  channel/1 -> ram_formatting/6(channel)
  header/1 -> ram_formatting/7(header)
  payload/1 -> ram_formatting/8(payload)
  ram_formatting/1(Out1) -> write_data/1
  Add1/1 -> Delay9/1
  Constant73/1 -> Add1/1
  Constant43/1 -> Delay1/1
  payload_len/1 -> Delay/1  "payload_len"
  Product/1 -> Delay8/1
  Delay9/1 -> Relational Operator/1, ram_size/1  "ram_size"
  Delay8/1 -> Add1/2

== system HDL_ieee_8021513/ofdm_symbol_sync/m_cox/calculate_P ==
  r(d) : Inport
  Add : Sum  OutDataTypeStr=Inherit: Same as first input
  Add1 : Sum
  Complex to Real-Imag : ComplexToRealImag
  Conjugate1 : Math  Operator=conj  SignedPower=on  OutputSignalType=complex  RndMeth=Zero
  Conjugate2 : Math  Operator=conj  SignedPower=on  OutputSignalType=complex  RndMeth=Zero
  Data Type Conversion1 : DataTypeConversion  OutDataTypeStr=CONST.dsp48A  SaturateOnIntegerOverflow=off  RndMeth=Floor
  Data Type Conversion2 : DataTypeConversion  OutDataTypeStr=CONST.dsp48B  SaturateOnIntegerOverflow=off  RndMeth=Floor
  Data Type Conversion3 : DataTypeConversion  OutDataTypeStr=CONST.dsp48A  SaturateOnIntegerOverflow=off  RndMeth=Floor
  Data Type Conversion4 : DataTypeConversion  OutDataTypeStr=CONST.dsp48B  SaturateOnIntegerOverflow=off  RndMeth=Floor
  Delay : Delay  DelayLength=1  InitialCondition=0  UseCircularBuffer=on
  Delay1 : Delay  DelayLength=(CONST.N+CONST.preambleCyclicPrefixLen)*5  InitialCondition=0  UseCircularBuffer=on
  Delay{3,5..7,11..12,14,16} (8 alike) : Delay  InitialCondition=0  UseCircularBuffer=on
  Delay13 : Delay  DelayLength=1  InitialCondition=0  UseCircularBuffer=on
  Delay2 : Delay  DelayLength=(CONST.N+CONST.preambleCyclicPrefixLen)*5  InitialCondition=0  UseCircularBuffer=on
  Delay4 : Delay  DelayLength=1  InitialCondition=0  UseCircularBuffer=on
  Product1 : Product
  Product2 : Product
  Subtract1 : Sum  Inputs=+-
  complex_multiplier : $bdroot/complex_multiplier  SystemSampleTime=-1  VariantActivationTime=update diagram  AllowFlexibleInterface=on  Latency=0  AutoFrameSizeCalculation=off
  complex_multiplier1 : $bdroot/complex_multiplier  SystemSampleTime=-1  VariantActivationTime=update diagram  AllowFlexibleInterface=on  Latency=0  AutoFrameSizeCalculation=off
  |P(d)|2 : Outport
  P(d) : Outport  Port=2  VectorParamsAs1DForOutWhenUnconnected=off
  wires:
  Product1/1 -> Delay12/1
  Delay7/1 -> Product1/2
  Data Type Conversion3/1 -> Delay6/1
  Data Type Conversion4/1 -> Delay7/1
  Delay6/1 -> Product1/1
  Complex to Real-Imag/1 -> Data Type Conversion3/1, Data Type Conversion4/1
  Data Type Conversion2/1 -> Delay5/1
  Delay5/1 -> Product2/2
  Data Type Conversion1/1 -> Delay14/1
  Subtract1/1 -> Add/1
  Conjugate2/1 -> complex_multiplier1/2
  Conjugate1/1 -> complex_multiplier/2
  Delay16/1 -> Delay3/1
  Delay14/1 -> Product2/1
  Delay13/1 -> |P(d)|2/1
  Add1/1 -> Delay13/1
  Delay11/1 -> Add1/2
  Delay12/1 -> Add1/1
  Product2/1 -> Delay11/1
  Complex to Real-Imag/2 -> Data Type Conversion1/1, Data Type Conversion2/1
  complex_multiplier/1 -> Subtract1/1
  complex_multiplier1/1 -> Subtract1/2
  Add/1 -> Delay/1  "acum"
  Delay2/1 -> Conjugate2/1  "r(d)"
  Delay1/1 -> Delay2/1, Conjugate1/1, complex_multiplier1/1  "r(d+L)"
  r(d)/1 -> Delay1/1, complex_multiplier/1  "r(d+2L)"
  Delay/1 -> Delay16/1, Complex to Real-Imag/1, Add/2  "P(d)"
  Delay3/1 -> Delay4/1
  Delay4/1 -> P(d)/1

== system HDL_ieee_8021513/ofdm_symbol_sync/m_cox/calculate_R ==
  r(d) : Inport
  Add : Sum  OutDataTypeStr=Inherit: Same as first input
  Add1 : Sum
  Complex to Real-Imag : ComplexToRealImag
  Data Type Conversion : DataTypeConversion  OutDataTypeStr=CONST.dsp48A  SaturateOnIntegerOverflow=off  RndMeth=Floor
  Data Type Conversion1 : DataTypeConversion  OutDataTypeStr=CONST.dsp48B  SaturateOnIntegerOverflow=off  RndMeth=Floor
  Delay : Delay  DelayLength=(CONST.N+CONST.preambleCyclicPrefixLen)*2*5  InitialCondition=0  UseCircularBuffer=on
  Delay1 : Delay  DelayLength=1  InitialCondition=0  UseCircularBuffer=on
  Delay{2..3,5..7,11..12} (7 alike) : Delay  InitialCondition=0  UseCircularBuffer=on
  Delay4 : Delay  DelayLength=1  InitialCondition=0  UseCircularBuffer=on
  Delay8 : Delay  DelayLength=1  InitialCondition=0  UseCircularBuffer=on
  Divide by 2 : hdlsllib/Logic and Bit Operations/Bit Shift  mode=Shift Right Arithmetic  N=1
  Product : Product
  Product1 : Product
  Product2 : Product
  Subtract : Sum  Inputs=+-
  Rf2 : Outport
  wires:
  Delay8/1 -> Delay/1, Subtract/1
  Divide by 2/1 -> Delay8/1
  Data Type Conversion1/1 -> Delay7/1
  Delay7/1 -> Product2/2
  Delay5/1 -> Product2/1
  Data Type Conversion/1 -> Delay5/1
  Delay6/1 -> Product1/1, Product1/2
  Delay3/1 -> Product/2, Product/1
  Complex to Real-Imag/2 -> Delay3/1
  Product/1 -> Delay11/1
  Add1/1 -> Delay4/1
  r(d)/1 -> Complex to Real-Imag/1  "P(d)"
  Delay11/1 -> Add1/2
  Complex to Real-Imag/1 -> Delay6/1
  Delay12/1 -> Add1/1
  Delay4/1 -> Divide by 2/1  "|r(d+2L)|2"
  Delay2/1 -> Rf2/1
  Subtract/1 -> Add/1
  Add/1 -> Delay1/1
  Delay1/1 -> Add/2, Data Type Conversion/1, Data Type Conversion1/1  "xxx"
  Delay/1 -> Subtract/2  "|r(d)|2"
  Product1/1 -> Delay12/1
  Product2/1 -> Delay2/1
